simulink model "dd_con"  (R2020a)
settings: Solver=VariableStepAuto  StartTime=0.0  StopTime=5  RelTol=1e-3
libraries: powerlib x10, powerlib_meascontrol x6
settings Model: Creator=abhin  LastModifiedBy=abhin

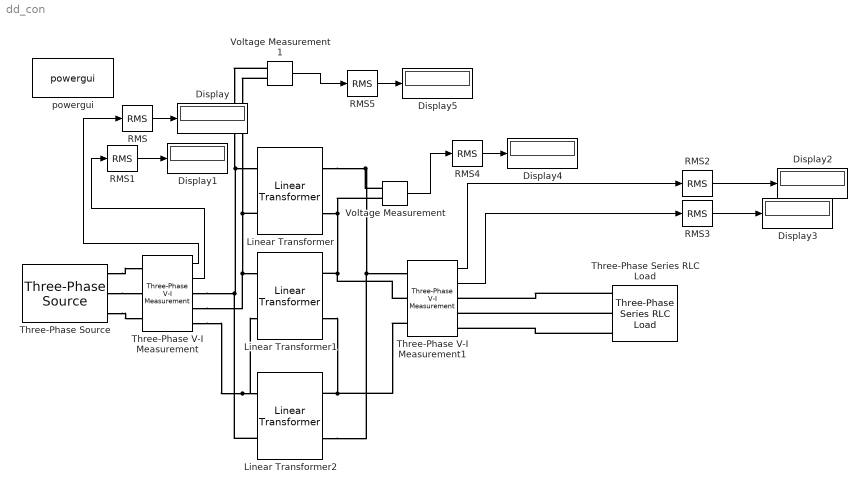
== system dd_con ==
  Display{,1..5} (6 alike) : Display
  Linear Transformer : powerlib/Elements/Linear Transformer  UNITS=SI  NominalPower=[ 250e6 50 ]  winding1=[400 4.3218 0.45856]  winding2=[200 0.7938 0.084225]  ThreeWindings=off  winding3=[3.15e+05 0.7938 0.084225]  RmLm=[1.0805e+06 2866]  Measurements=None  DataType=on
  Linear Transformer1 : powerlib/Elements/Linear Transformer  UNITS=SI  NominalPower=[ 250e6 50 ]  winding1=[400 1.28e-06 1.6297e-07]  winding2=[200 3.2e-07 4.0744e-08]  ThreeWindings=off  winding3=[3.15e+05 0.7938 0.10107]  RmLm=[0.32 0.0010186]  Measurements=None  DataType=on
  Linear Transformer2 : powerlib/Elements/Linear Transformer  UNITS=SI  NominalPower=[ 250e6 50 ]  winding1=[400 1.28e-06 1.6297e-07]  winding2=[200 2e-08 2.5465e-09]  ThreeWindings=off  winding3=[3.15e+05 0.7938 0.10107]  RmLm=[0.32 0.0010186]  Measurements=None  DataType=on
  RMS{,1..5} (6 alike) : powerlib_meascontrol/Measurements/RMS  TrueRMS=on  Freq=50  RMSInit=120  Ts=0
  Three-Phase Series RLC Load : powerlib/Elements/Three-Phase Series RLC Load  LConnTagsString=A|B|C  Configuration=Y (grounded)  NominalVoltage=1000  Vabc=[1e3 1e3 1e3]  Vabcp=[1e3 1e3 1e3]  NominalFrequency=50  UnbalancedPower=off  ActivePower=10e7  InductivePower=0  CapacitivePower=0  Pabc=[10e3 9e3 11e3]  QLabc=[100 90 110]  QCabc=[100 90 110]  Pabcp=[10e3 9e3 11e3]  QLabcp=[100 90 110]  QCabcp=[100 90 110]  Measurements=None  LoadType=constant Z
  Three-Phase V-I Measurement : powerlib/Measurements/Three-Phase V-I Measurement  VoltageMeasurement=phase-to-ground  SetLabelV=off  LabelV=Vabc  Vpu=off  VpuLL=off  CurrentMeasurement=yes  SetLabelI=off  LabelI=Iabc  Ipu=off  Pbase=100e6  Vbase=500e3  OutputType=Complex  PhasorSimulation=off  PSBequivalent=0
  Three-Phase V-I Measurement1 : powerlib/Measurements/Three-Phase V-I Measurement  VoltageMeasurement=phase-to-ground  SetLabelV=off  LabelV=Vabc  Vpu=off  VpuLL=off  CurrentMeasurement=yes  SetLabelI=off  LabelI=Iabc  Ipu=off  Pbase=100e6  Vbase=500e3  OutputType=Complex  PhasorSimulation=off  PSBequivalent=0
  Three-Phase Source : powerlib/Electrical Sources/Three-Phase Source  InternalConnection=Yg  VoltagePhases=off  Voltage=400  PhaseAngle=0  Voltage_phases=[25e3 25e3 25e3]/sqrt(3)  PhaseAngles_phases=[0 -120 +120]  Frequency=50  NonIdealSource=off  SpecifyImpedance=off  Resistance=0.8929  Inductance=0  ShortCircuitLevel=100e6  BaseVoltage=25e3  XRratio=7  BusType=swing  Pref=10e3  Qref=0  Prefabc=[10e3, 10e3, 10e3]  Qrefabc=[0, 0, 0]  Qmin=-inf  Qmax=inf
  Voltage Measurement : powerlib/Measurements/Voltage Measurement  PhasorSimulation=off  OutputType=Complex  PSBequivalent=0
  Voltage Measurement1 : powerlib/Measurements/Voltage Measurement  PhasorSimulation=off  OutputType=Complex  PSBequivalent=0
  powergui : powerlib/powergui  Priority=1  SimulationMode=Discrete  SampleTime=50e-6  frequency=60  Iterations=50  frequencyindice=50  Pbase=100e6  ErrMax=1e-4  UnitsV=kV  UnitsW=MW  buscounter=0  FunctionMessages=off  echomessages=off  EnableUseOfTLC=off  CurrentSourceSwitches=off  DisableSnubberDevices=off  DisableRonSwitches=off  DisableVfSwitches=off  DisplayEquations=off  AutomaticDiscreteSolvers=off  SolverType=Tustin/Backward Euler (TBE)  Interpol=off  ExternalGateDelay=off  methode=off  Ts=100  x0status=blocks  SPID=on  SwTol=0  HookPort=off  NonlinearTolerance=1e-4  nMaxIteration=100  ContinueOnMaxIteration=off  RestoreLinks=warning  ResistiveCurrentMeasurement=off  Frange=[0:2:500]  Ylog=off  Xlog=on  ShowGrid=off  save=off  variable=ZData  structure=0  ZoomFFT=off  StartTime=0.0  cycles=1  DisplayStyle=1  fundamental=60  FreqAxis=off  MaxFrequency=1000  frequencyindicesteady=1  RmsSteady=1  display=off
  wires:
  RMS/1 -> Display/1
  RMS1/1 -> Display1/1
  RMS2/1 -> Display2/1
  RMS3/1 -> Display3/1
  Three-Phase V-I Measurement/1 -> RMS/1
  Three-Phase V-I Measurement/2 -> RMS1/1
  Three-Phase V-I Measurement1/1 -> RMS2/1
  Three-Phase V-I Measurement1/2 -> RMS3/1
  RMS4/1 -> Display4/1
  Voltage Measurement/1 -> RMS4/1
  RMS5/1 -> Display5/1
  Voltage Measurement1/1 -> RMS5/1
  connections:
  Three-Phase Source/RConn1 -- Three-Phase V-I Measurement/LConn1
  Three-Phase Source/RConn2 -- Three-Phase V-I Measurement/LConn2
  Three-Phase Source/RConn3 -- Three-Phase V-I Measurement/LConn3
  Linear Transformer2/LConn1 -- Linear Transformer1/LConn2 -- Three-Phase V-I Measurement/RConn3
  Linear Transformer/LConn2 -- Voltage Measurement1/LConn2 -- Three-Phase V-I Measurement/RConn2 -- Linear Transformer1/LConn1
  Three-Phase V-I Measurement/RConn1 -- Linear Transformer2/LConn2 -- Linear Transformer/LConn1 -- Voltage Measurement1/LConn1
  Linear Transformer/RConn1 -- Voltage Measurement/LConn1 -- Linear Transformer2/RConn2 -- Three-Phase V-I Measurement1/LConn1
  Linear Transformer/RConn2 -- Three-Phase V-I Measurement1/LConn2 -- Linear Transformer1/RConn1 -- Voltage Measurement/LConn2
  Linear Transformer1/RConn2 -- Three-Phase V-I Measurement1/LConn3 -- Linear Transformer2/RConn1
  Three-Phase Series RLC Load/LConn3 -- Three-Phase V-I Measurement1/RConn3
  Three-Phase Series RLC Load/LConn2 -- Three-Phase V-I Measurement1/RConn2
  Three-Phase Series RLC Load/LConn1 -- Three-Phase V-I Measurement1/RConn1
